simulink model "SAFECOPYFOC_Motor_Control_Hardware"  (R2025b)
settings: Solver=FixedStepDiscrete  StartTime=0.0  StopTime=inf  FixedStep=50e-6  MaxStep=1e-4  RelTol=1e-3  EnableMultiTasking=on
values from neighbouring files (symbols this model uses):
  Ki_d = R   * omega_c    [VirtualSpeedDynoParams.m]
  Ki_q = R   * omega_c    [VirtualSpeedDynoParams.m]
  Kp_d = L_d * omega_c    [VirtualSpeedDynoParams.m]
  Kp_q = L_q * omega_c    [VirtualSpeedDynoParams.m]
  L_d = motor.L_phase_H    [VirtualSpeedDynoParams.m]
  L_q = motor.L_phase_H    [VirtualSpeedDynoParams.m]
  lambda = motor.lambda_Wb    [VirtualSpeedDynoParams.m]
  p = motor.pole_pairs    [VirtualSpeedDynoParams.m]
  V_bat = motor.bus_voltage_V    [VirtualSpeedDynoParams.m]
undefined symbols (not defined in the file or in its folder): bit, Down, GPTRIP1SEL, GPTRIP2SEL, target, TZ1, TZ2, Up
libraries: c2802xlib x5, c280xlib x3, slpidlib x3, c2806xlib x2, eeTransforms x2, simulink x1

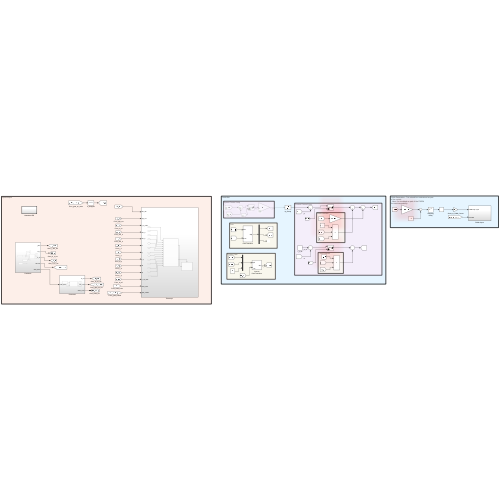
[thumbnail: Simulink's stored preview of the top-level diagram]
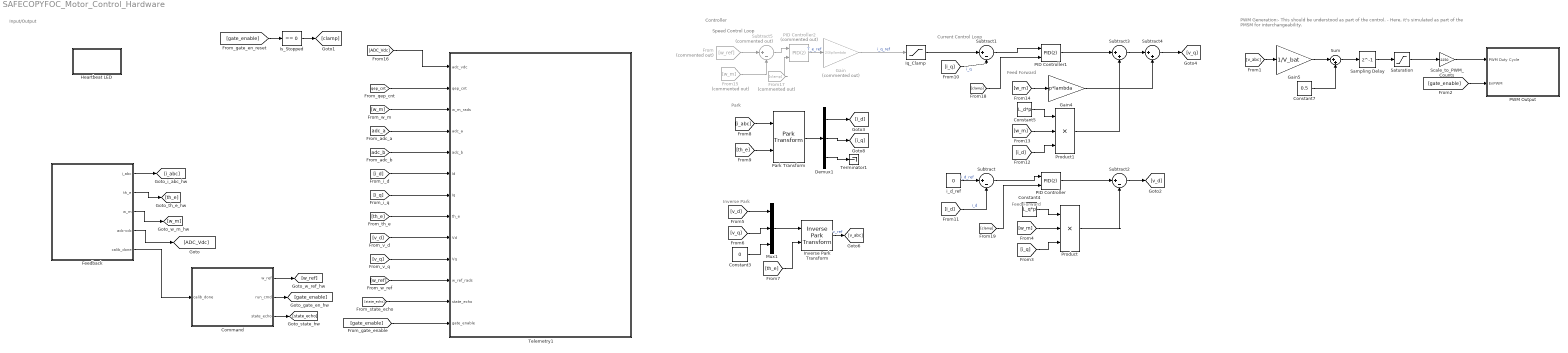
== system SAFECOPYFOC_Motor_Control_Hardware ==
  note: Feed Forward
  note: Feed Forward
  note: Current Control Loop
  note: Speed Control Loop
  note: Input/Output
  note: Park
  note: Inverse Park
  note: PWM Generation:- This should be understood as part
      | of the control.
      | - Here, it's simulated as part of the PMSM
      | for interchangeability.
  note: Controller
  Command : Subsystem
  Constant3 : Constant  Value=0  OutDataTypeStr=single
  Constant4 : Constant  Value=L_q*p  OutDataTypeStr=single
  Constant5 : Constant  Value=L_d*p  OutDataTypeStr=single
  Constant7 : Constant  Value=0.5  OutDataTypeStr=single
  Demux1 : Demux  Outputs=3
  Feedback : Subsystem
  From : From  Commented=on  GotoTag=w_ref
  From15 : From  Commented=on  GotoTag=w_m
  From17 : From  Commented=on  GotoTag=clamp
  Gain : Gain  Commented=on  Gain=2/3/p/lambda
  Gain4 : Gain  Gain=p*lambda
  Gain5 : Gain  Gain=1/V_bat
  Heartbeat LED : Subsystem  TreatAsAtomicUnit=on
  Inverse Park Transform : eeTransforms/Inverse Park Transform  AxisAlignment=D-axis  PowerInvariant=off
  Iq_Clamp : Saturate
  Is_Stopped : simulink/Logic and Bit Operations/Compare To Zero  relop===  OutDataTypeStr=boolean
  Mux1 : Mux  Inputs=3
  PID Controller : slpidlib/PID Controller  Controller=PID  Form=Parallel  TimeDomain=Discrete-time  UseExternalTs=off  SampleTime=50e-6  IntegratorMethod=Forward Euler  FilterMethod=Forward Euler  ControllerParametersSource=internal  P=Kp_d  I=Ki_d  UseKiTs=off  D=0  UseExternalDerivativeSource=off  N=100  UseFilter=on  TunerSelectOption=Transfer Function Based (PID Tuner App)  InitialConditionSource=internal  InitialConditionForIntegrator=0  InitialConditionForFilter=0  DifferentiatorICPrevScaledInput=0  ExternalReset=level  TrackingMode=off  Kt=1  LimitOutput=on  SatLimitsSource=internal  UpperSaturationLimit=V_bat/sqrt(3)  LowerSaturationLimit=-(V_bat/sqrt(3))  LinearizeAsGain=on  AntiWindupMode=clamping  Kb=1  LimitIntegrator=off  UpperIntegratorSaturationLimit=inf  LowerIntegratorSaturationLimit=-inf  POutMin=[]  POutMax=[]  IOutMin=[]  IOutMax=[]  DOutMin=[]  DOutMax=[]  NOutMin=[]  NOutMax=[]  SumOutMin=[]  SumOutMax=[]  SaturationOutMin=[]  SaturationOutMax=[]  PParamMin=[]  PParamMax=[]  IParamMin=[]  IParamMax=[]  DParamMin=[]  DParamMax=[]  NParamMin=[]  NParamMax=[]  KbParamMin=[]  KbParamMax=[]  KtParamMin=[]  KtParamMax=[]  KbOutMin=[]  KbOutMax=[]  KtOutMin=[]  KtOutMax=[]  IntegratorOutMin=[]  IntegratorOutMax=[]  FilterOutMin=[]  FilterOutMax=[]  SumI1OutMin=[]  SumI1OutMax=[]  SumI2OutMin=[]  SumI2OutMax=[]  SumI3OutMin=[]  SumI3OutMax=[]  SumI4OutMin=[]  SumI4OutMax=[]  SumDOutMin=[]  SumDOutMax=[]  DifferentiatorOutMin=[]  DifferentiatorOutMax=[]  FilterDiffOutCoefMin=[]  FilterDiffOutCoefMax=[]  ReciprocalOutMin=[]  ReciprocalOutMax=[]  SumDenOutMin=[]  SumDenOutMax=[]  SumNumOutMin=[]  SumNumOutMax=[]  DivideOutMin=[]  DivideOutMax=[]  UdiffTsProdOutMin=[]  UdiffTsProdOutMax=[]  NTsProdOutMin=[]  NTsProdOutMax=[]  UintegralTsProdOutMin=[]  UintegralTsProdOutMax=[]  UngainTsProdOutMin=[]  UngainTsProdOutMax=[]  ClampingZeroOutDataTypeStr=Inherit: Inherit via back propagation  ClampingZeroOutMin=[]  ClampingZeroOutMax=[]  FilterDenConstantOutDataTypeStr=Inherit: Inherit via back propagation  FilterDenConstantOutMin=[]  FilterDenConstantOutMax=[]  PCopyOutDataTypeStr=Inherit: Inherit via back propagation  PCopyOutMin=[]  PCopyOutMax=[]  NCopyOutDataTypeStr=Inherit: Inherit via back propagation  NCopyOutMin=[]  NCopyOutMax=[]  IntegratorContinuousStateAttributes=''  IntegratorStateMustResolveToSignalObject=off  IntegratorRTWStateStorageClass=Auto  FilterContinuousStateAttributes=''  FilterStateMustResolveToSignalObject=off  FilterRTWStateStorageClass=Auto  ParallelPVariant=InternalParameters  IdealPVariant=Disabled  IVariant=InternalParameters  DVariant=InternalParameters  IntegratorVariant=Discrete  SatVariant=Enabled  AWVariant=DiscClampingParallel  PCopyVariant=Disabled  TRVariant=Disabled  FdbkBlocksVariant=Forward  IdealPFdbkVariant=Disabled  SatFdbkVariant=Disabled  DerivativeFilterVariant=ForwardEulerFilter  NVariant=InternalParameters  NCopyVariant=Disabled  FilterICVariant=InternalICsFilter  IntegratorICVariant=InternalICs  ExternalResetVariant=ExternalReset  TRSumVariant=Passthrough  SumFdbkVariant=Disabled  SumVariant=Sum_PID  TsampFilterVariant=InternalTs  TsampNgainVariant=Passthrough  TsampIntegralVariant=Disabled_SignalSpec  ExternalSaturationOutDataTypeStr=Inherit: Same as second input  DerivativeSourceVariant=ErrorSignal  PreIntVariant=InternalPreInt
  PID Controller1 : slpidlib/PID Controller  Controller=PID  Form=Parallel  TimeDomain=Discrete-time  UseExternalTs=off  SampleTime=50e-6  IntegratorMethod=Forward Euler  FilterMethod=Forward Euler  ControllerParametersSource=internal  P=Kp_q  I=Ki_q  UseKiTs=off  D=0  UseExternalDerivativeSource=off  N=100  UseFilter=on  TunerSelectOption=Transfer Function Based (PID Tuner App)  InitialConditionSource=internal  InitialConditionForIntegrator=0  InitialConditionForFilter=0  DifferentiatorICPrevScaledInput=0  ExternalReset=level  TrackingMode=off  Kt=1  LimitOutput=on  SatLimitsSource=internal  UpperSaturationLimit=V_bat/sqrt(3)  LowerSaturationLimit=-(V_bat/sqrt(3))  LinearizeAsGain=on  AntiWindupMode=clamping  Kb=1  LimitIntegrator=off  UpperIntegratorSaturationLimit=inf  LowerIntegratorSaturationLimit=-inf  POutMin=[]  POutMax=[]  IOutMin=[]  IOutMax=[]  DOutMin=[]  DOutMax=[]  NOutMin=[]  NOutMax=[]  SumOutMin=[]  SumOutMax=[]  SaturationOutMin=[]  SaturationOutMax=[]  PParamMin=[]  PParamMax=[]  IParamMin=[]  IParamMax=[]  DParamMin=[]  DParamMax=[]  NParamMin=[]  NParamMax=[]  KbParamMin=[]  KbParamMax=[]  KtParamMin=[]  KtParamMax=[]  KbOutMin=[]  KbOutMax=[]  KtOutMin=[]  KtOutMax=[]  IntegratorOutMin=[]  IntegratorOutMax=[]  FilterOutMin=[]  FilterOutMax=[]  SumI1OutMin=[]  SumI1OutMax=[]  SumI2OutMin=[]  SumI2OutMax=[]  SumI3OutMin=[]  SumI3OutMax=[]  SumI4OutMin=[]  SumI4OutMax=[]  SumDOutMin=[]  SumDOutMax=[]  DifferentiatorOutMin=[]  DifferentiatorOutMax=[]  FilterDiffOutCoefMin=[]  FilterDiffOutCoefMax=[]  ReciprocalOutMin=[]  ReciprocalOutMax=[]  SumDenOutMin=[]  SumDenOutMax=[]  SumNumOutMin=[]  SumNumOutMax=[]  DivideOutMin=[]  DivideOutMax=[]  UdiffTsProdOutMin=[]  UdiffTsProdOutMax=[]  NTsProdOutMin=[]  NTsProdOutMax=[]  UintegralTsProdOutMin=[]  UintegralTsProdOutMax=[]  UngainTsProdOutMin=[]  UngainTsProdOutMax=[]  ClampingZeroOutDataTypeStr=Inherit: Inherit via back propagation  ClampingZeroOutMin=[]  ClampingZeroOutMax=[]  FilterDenConstantOutDataTypeStr=Inherit: Inherit via back propagation  FilterDenConstantOutMin=[]  FilterDenConstantOutMax=[]  PCopyOutDataTypeStr=Inherit: Inherit via back propagation  PCopyOutMin=[]  PCopyOutMax=[]  NCopyOutDataTypeStr=Inherit: Inherit via back propagation  NCopyOutMin=[]  NCopyOutMax=[]  IntegratorContinuousStateAttributes=''  IntegratorStateMustResolveToSignalObject=off  IntegratorRTWStateStorageClass=Auto  FilterContinuousStateAttributes=''  FilterStateMustResolveToSignalObject=off  FilterRTWStateStorageClass=Auto  ParallelPVariant=InternalParameters  IdealPVariant=Disabled  IVariant=InternalParameters  DVariant=InternalParameters  IntegratorVariant=Discrete  SatVariant=Enabled  AWVariant=DiscClampingParallel  PCopyVariant=Disabled  TRVariant=Disabled  FdbkBlocksVariant=Forward  IdealPFdbkVariant=Disabled  SatFdbkVariant=Disabled  DerivativeFilterVariant=ForwardEulerFilter  NVariant=InternalParameters  NCopyVariant=Disabled  FilterICVariant=InternalICsFilter  IntegratorICVariant=InternalICs  ExternalResetVariant=ExternalReset  TRSumVariant=Passthrough  SumFdbkVariant=Disabled  SumVariant=Sum_PID  TsampFilterVariant=InternalTs  TsampNgainVariant=Passthrough  TsampIntegralVariant=Disabled_SignalSpec  ExternalSaturationOutDataTypeStr=Inherit: Same as second input  DerivativeSourceVariant=ErrorSignal  PreIntVariant=InternalPreInt
  PID Controller2 : slpidlib/PID Controller  Commented=on  Controller=PID  Form=Parallel  TimeDomain=Discrete-time  UseExternalTs=off  SampleTime=50e-6  IntegratorMethod=Forward Euler  FilterMethod=Forward Euler  ControllerParametersSource=internal  P=2.5  I=1.5  UseKiTs=off  D=0  UseExternalDerivativeSource=off  N=100  UseFilter=on  TunerSelectOption=Transfer Function Based (PID Tuner App)  InitialConditionSource=internal  InitialConditionForIntegrator=0  InitialConditionForFilter=0  DifferentiatorICPrevScaledInput=0  ExternalReset=level  TrackingMode=off  Kt=1  LimitOutput=on  SatLimitsSource=internal  UpperSaturationLimit=60  LowerSaturationLimit=-60  LinearizeAsGain=on  AntiWindupMode=clamping  Kb=1  LimitIntegrator=off  UpperIntegratorSaturationLimit=inf  LowerIntegratorSaturationLimit=-inf  POutMin=[]  POutMax=[]  IOutMin=[]  IOutMax=[]  DOutMin=[]  DOutMax=[]  NOutMin=[]  NOutMax=[]  SumOutMin=[]  SumOutMax=[]  SaturationOutMin=[]  SaturationOutMax=[]  PParamMin=[]  PParamMax=[]  IParamMin=[]  IParamMax=[]  DParamMin=[]  DParamMax=[]  NParamMin=[]  NParamMax=[]  KbParamMin=[]  KbParamMax=[]  KtParamMin=[]  KtParamMax=[]  KbOutMin=[]  KbOutMax=[]  KtOutMin=[]  KtOutMax=[]  IntegratorOutMin=[]  IntegratorOutMax=[]  FilterOutMin=[]  FilterOutMax=[]  SumI1OutMin=[]  SumI1OutMax=[]  SumI2OutMin=[]  SumI2OutMax=[]  SumI3OutMin=[]  SumI3OutMax=[]  SumI4OutMin=[]  SumI4OutMax=[]  SumDOutMin=[]  SumDOutMax=[]  DifferentiatorOutMin=[]  DifferentiatorOutMax=[]  FilterDiffOutCoefMin=[]  FilterDiffOutCoefMax=[]  ReciprocalOutMin=[]  ReciprocalOutMax=[]  SumDenOutMin=[]  SumDenOutMax=[]  SumNumOutMin=[]  SumNumOutMax=[]  DivideOutMin=[]  DivideOutMax=[]  UdiffTsProdOutMin=[]  UdiffTsProdOutMax=[]  NTsProdOutMin=[]  NTsProdOutMax=[]  UintegralTsProdOutMin=[]  UintegralTsProdOutMax=[]  UngainTsProdOutMin=[]  UngainTsProdOutMax=[]  ClampingZeroOutDataTypeStr=Inherit: Inherit via back propagation  ClampingZeroOutMin=[]  ClampingZeroOutMax=[]  FilterDenConstantOutDataTypeStr=Inherit: Inherit via back propagation  FilterDenConstantOutMin=[]  FilterDenConstantOutMax=[]  PCopyOutDataTypeStr=Inherit: Inherit via back propagation  PCopyOutMin=[]  PCopyOutMax=[]  NCopyOutDataTypeStr=Inherit: Inherit via back propagation  NCopyOutMin=[]  NCopyOutMax=[]  IntegratorContinuousStateAttributes=''  IntegratorStateMustResolveToSignalObject=off  IntegratorRTWStateStorageClass=Auto  FilterContinuousStateAttributes=''  FilterStateMustResolveToSignalObject=off  FilterRTWStateStorageClass=Auto  ParallelPVariant=InternalParameters  IdealPVariant=Disabled  IVariant=InternalParameters  DVariant=InternalParameters  IntegratorVariant=Discrete  SatVariant=Enabled  AWVariant=DiscClampingParallel  PCopyVariant=Disabled  TRVariant=Disabled  FdbkBlocksVariant=Forward  IdealPFdbkVariant=Disabled  SatFdbkVariant=Disabled  DerivativeFilterVariant=ForwardEulerFilter  NVariant=InternalParameters  NCopyVariant=Disabled  FilterICVariant=InternalICsFilter  IntegratorICVariant=InternalICs  ExternalResetVariant=ExternalReset  TRSumVariant=Passthrough  SumFdbkVariant=Disabled  SumVariant=Sum_PID  TsampFilterVariant=InternalTs  TsampNgainVariant=Passthrough  TsampIntegralVariant=Disabled_SignalSpec  ExternalSaturationOutDataTypeStr=Inherit: Same as second input  DerivativeSourceVariant=ErrorSignal  PreIntVariant=InternalPreInt
  PWM Output : Subsystem
  Park Transform : eeTransforms/Park Transform  AxisAlignment=D-axis  PowerInvariant=off
  Product : Product  Inputs=3
  Product1 : Product  Inputs=3
  Sampling Delay : Delay  DelayLength=1
  Saturation : Saturate  UpperLimit=1  LowerLimit=0
  Scale_to_PWM_Counts : Gain  Gain=2250
  Subtract : Sum  Inputs=|+-
  Subtract1 : Sum  Inputs=|+-
  Subtract2 : Sum  Inputs=|+-
  Subtract3 : Sum  Inputs=|++
  Subtract4 : Sum  Inputs=|++
  Subtract5 : Sum  Commented=on  Inputs=|+-
  Sum : Sum  Inputs=|++
  Telemetry1 : Subsystem
  Terminator1 : Terminator
  i_d_ref : Constant  Value=0  OutDataTypeStr=single
  wires:
  [qep_cnt] -> Telemetry1/2(qep_cnt)
  [w_m] -> Telemetry1/3(w_m_rads)
  [adc_a] -> Telemetry1/4(adc_a)
  [adc_b] -> Telemetry1/5(adc_b)
  [i_d] -> Telemetry1/6(Id)
  [i_q] -> Telemetry1/7(Iq)
  [th_e] -> Telemetry1/8(th_e)
  [v_d] -> Telemetry1/9(Vd)
  [v_q] -> Telemetry1/10(Vq)
  [w_ref] -> Telemetry1/11(w_ref_rads)
  [state_echo] -> Telemetry1/12(state_echo)
  [gate_enable] -> Telemetry1/13(gate_enable)
  Command/1(w_ref) -> [w_ref]
  Command/2(run_cmd) -> [gate_enable]
  Command/3(state_echo) -> [state_echo]
  Feedback/5(calib_done) -> Command/1(calib_done)
  Feedback/3(w_m) -> [w_m]
  Feedback/2(th_e) -> [th_e]
  Feedback/1(i_abc) -> [i_abc]
  From/1 -> Subtract5/1
  From15/1 -> Subtract5/2
  Subtract5/1 -> PID Controller2/1
  PID Controller2/1 -> Gain/1  "T_e_ref"
  Gain/1 -> Iq_Clamp/1  "i_q_ref"
  Iq_Clamp/1 -> Subtract1/1
  [i_q] -> Subtract1/2  "i_q"
  Subtract1/1 -> PID Controller1/1
  PID Controller1/1 -> Subtract3/1
  Product1/1 -> Subtract3/2
  [w_m] -> Gain4/1
  Constant5/1 -> Product1/1
  [w_m] -> Product1/2
  [i_d] -> Product1/3
  Gain4/1 -> Subtract4/2
  Subtract3/1 -> Subtract4/1
  Subtract4/1 -> [v_q]
  [v_abc] -> Gain5/1
  Gain5/1 -> Sum/1
  Constant7/1 -> Sum/2
  Sum/1 -> Sampling Delay/1
  Sampling Delay/1 -> Saturation/1
  Saturation/1 -> Scale_to_PWM_Counts/1
  Scale_to_PWM_Counts/1 -> PWM Output/1(PWM Duty Cycle)
  [gate_enable] -> PWM Output/2(EnPWM)
  i_d_ref/1 -> Subtract/1  "i_d_ref"
  [i_d] -> Subtract/2  "i_d"
  Subtract/1 -> PID Controller/1
  PID Controller/1 -> Subtract2/1
  Product/1 -> Subtract2/2
  Subtract2/1 -> [v_d]
  Constant4/1 -> Product/1
  [w_m] -> Product/2
  [i_q] -> Product/3
  Inverse Park Transform/1 -> [v_abc]  "v_ref"
  Mux1/1 -> Inverse Park Transform/1
  [th_e] -> Inverse Park Transform/2
  Constant3/1 -> Mux1/3
  [v_q] -> Mux1/2
  [v_d] -> Mux1/1
  [th_e] -> Park Transform/2
  [i_abc] -> Park Transform/1
  Demux1/1 -> [i_d]
  Demux1/2 -> [i_q]
  Demux1/3 -> Terminator1/1
  Park Transform/1 -> Demux1/1
  Feedback/4(adc-vdc) -> [ADC_Vdc]
  [ADC_Vdc] -> Telemetry1/1(adc_vdc)
  [gate_enable] -> Is_Stopped/1
  Is_Stopped/1 -> [clamp]
  From17/1 -> PID Controller2/2
  [clamp] -> PID Controller1/2
  [clamp] -> PID Controller/2

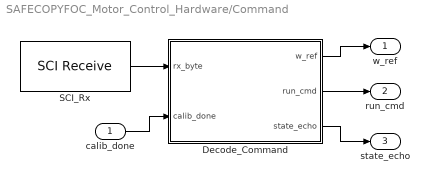
== system SAFECOPYFOC_Motor_Control_Hardware/Command ==
  calib_done : Inport
  Decode_Command : MATLAB Function  TreatAsAtomicUnit=on
  SCI_Rx : c280xlib/SCI Receive  sciModule=A  dataHead=''  headerCheckMaxCount=16  dataTail=''  dataType=uint8  dataLenOptions=Length via dialog  dataDim=1  maxDataLength=1  initValue=0  errOption=Output custom value  errValue=0  sampleTime=-1  blockingMode=off  timeOut=0.019444  outputStatus=off
  w_ref : Outport
  run_cmd : Outport  Port=2
  state_echo : Outport  Port=3
  wires:
  Decode_Command/3(state_echo) -> state_echo/1
  SCI_Rx/1 -> Decode_Command/1(rx_byte)
  calib_done/1 -> Decode_Command/2(calib_done)
  Decode_Command/1(w_ref) -> w_ref/1
  Decode_Command/2(run_cmd) -> run_cmd/1

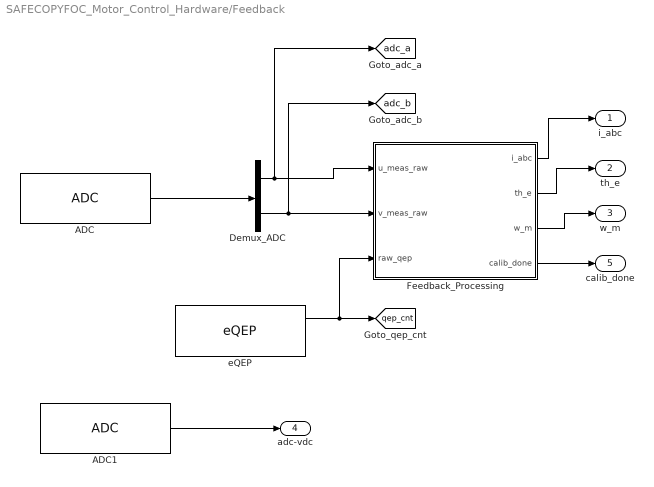
== system SAFECOPYFOC_Motor_Control_Hardware/Feedback ==
  ADC : c2802xlib/ADC  blkParamProc=C2000  ADCModule=1  samplingMode=Simultaneous sample mode  ADCResolution=12-bit (Single-ended input)  ADC29xResolution=12-bit  ADCMode=Single-ended input  useSOC1=SOC0  useSOC2=SOC0_SOC1  SOCAcquisitionWindow=7  SOCTriggerSource=Software  SOCInterruptTrigger=No ADCINT  Ts=-1  dType=uint16  postInterrupt=on  interruptSel=ADCINT1  ADCINTContinuous=on  endma=off  chdma=1  conv1=ADCINA0  conv2=ADCINA3 and ADCINB3  conv1_Type4=ADCIN0  conv2_Type4=ADCIN0 and ADCIN1
  ADC1 : c2802xlib/ADC  blkParamProc=C2000  ADCModule=1  samplingMode=Simultaneous sample mode  ADCResolution=12-bit (Single-ended input)  ADC29xResolution=12-bit  ADCMode=Single-ended input  useSOC1=SOC2  useSOC2=SOC2_SOC3  SOCAcquisitionWindow=7  SOCTriggerSource=Software  SOCInterruptTrigger=No ADCINT  Ts=-1  dType=uint16  postInterrupt=off  interruptSel=ADCINT1  ADCINTContinuous=on  endma=off  chdma=1  conv1=ADCINB7  conv2=ADCINA1 and ADCINB1  conv1_Type4=ADCIN0  conv2_Type4=ADCIN0 and ADCIN1
  Demux_ADC : Demux  Outputs=2
  Feedback_Processing : MATLAB Function  TreatAsAtomicUnit=on
  eQEP : c280xlib/eQEP  useModule=eQEP1  pcInputmode=Quadrature-count  externalClockrate=2x resolution: Count the rising/falling edge  swapPolarityselection=Clockwise  qdfOutputport=off  qapPolarityselection=off  qbpPolarityselection=off  qipPolarityselection=off  qspPolarityselection=off  igatePolarityselection=off  sampleTime=-1  pcOutputport=on  pcMaximumvalue=4*1024 - 1  indexInitializationcheck=off  indexInitializationevent=Falling edge  strobeInitializationcheck=off  strobeInitializationevent=Rising edge  softwareInitializationcheck=off  softwareInitializationsource=Set to init value at start up  softwareInitializationmode=on  pcInitialvalue=0  pcResetmode=Reset on the first index event  ieloutputport=on  indexEventlatch=Rising edge  seloutputport=off  strobeEventlatch=Rising edge  pcefOutputport=off  enableEqepcapture=off  qctmrOutputport=off  qcprdOutputport=off  captureTimerprescaler=128  upEventprescaler=128  overflowErrorflag=off  directionErrorflag=off  captureTimerposition=On position counter read  unitTimerperiod=100000000  captureTimerlatch=off  capturePeriodlatch=off  positionCounterlatch=off  soenPolarityselection=off  spselPolarityselection=Index pin is used for sync output  compareValuesource=Specify via dialog  shadowMode=Load on QPOSCNT=0  compareValue=4294967295  syncOutputwidth=1  polaritySyncoutput=Active high  watchdogEnable=off  watchdogTimer=65535  outport1Datatype=auto  outport2Datatype=auto  outport3Datatype=auto  outport4Datatype=auto  outport5Datatype=auto  outport6Datatype=auto  outport7Datatype=auto  outport8Datatype=auto  outport9Datatype=auto  outport10Datatype=auto  outport11Datatype=auto  outport12Datatype=auto  eqepinterrupt_pce=off  eqepinterrupt_qpe=off  eqepinterrupt_qdc=off  eqepinterrupt_wto=off  eqepinterrupt_pcu=off  eqepinterrupt_pco=off  eqepinterrupt_pcr=off  eqepinterrupt_pcm=off  eqepinterrupt_sel=off  eqepinterrupt_iel=off  eqepinterrupt_uto=off  pheOutputport=off  watchdogOutputport=off  outport13Datatype=auto  outport14Datatype=auto
  i_abc : Outport
  th_e : Outport  Port=2
  w_m : Outport  Port=3
  adc-vdc : Outport  Port=4
  calib_done : Outport  Port=5
  tag scope: adc_a=global, adc_b=global, qep_cnt=global
  wires:
  Demux_ADC/1 -> Feedback_Processing/1(u_meas_raw), [adc_a]
  ADC/1 -> Demux_ADC/1
  Feedback_Processing/2(th_e) -> th_e/1
  eQEP/1 -> [qep_cnt], Feedback_Processing/3(raw_qep)
  Demux_ADC/2 -> Feedback_Processing/2(v_meas_raw), [adc_b]
  Feedback_Processing/1(i_abc) -> i_abc/1
  Feedback_Processing/4(calib_done) -> calib_done/1
  Feedback_Processing/3(w_m) -> w_m/1
  ADC1/1 -> adc-vdc/1

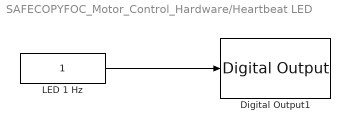
== system SAFECOPYFOC_Motor_Control_Hardware/Heartbeat LED ==
  Digital Output1 : c2806xlib/Digital Output  GPIO_Number=GPIO32~GPIO39  GPIO_Bit0=off  GPIO_BIT0_Toggle=off  GPIO_Bit1=off  GPIO_BIT1_Toggle=off  GPIO_Bit2=on  GPIO_BIT2_Toggle=on  GPIO_Bit3=off  GPIO_BIT3_Toggle=off  GPIO_Bit4=off  GPIO_BIT4_Toggle=off  GPIO_Bit5=off  GPIO_BIT5_Toggle=off  GPIO_Bit6=off  GPIO_BIT6_Toggle=off  GPIO_Bit7=off  GPIO_BIT7_Toggle=off
  LED 1 Hz : Constant  OutDataTypeStr=uint16  SampleTime=0.5
  wires:
  LED 1 Hz/1 -> Digital Output1/1

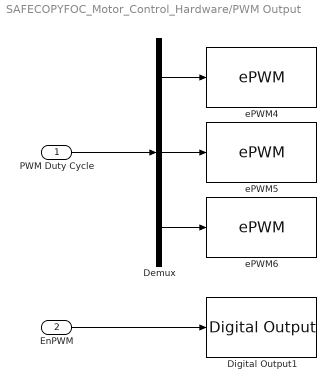
== system SAFECOPYFOC_Motor_Control_Hardware/PWM Output ==
  PWM Duty Cycle : Inport
  EnPWM : Inport  Port=2
  Demux : Demux  Outputs=3
  Digital Output1 : c2806xlib/Digital Output  GPIO_Number=GPIO50~GPIO55  GPIO_Bit0=off  GPIO_BIT0_Toggle=off  GPIO_Bit1=off  GPIO_BIT1_Toggle=off  GPIO_Bit2=on  GPIO_BIT2_Toggle=off  GPIO_Bit3=off  GPIO_BIT3_Toggle=off  GPIO_Bit4=off  GPIO_BIT4_Toggle=off  GPIO_Bit5=off  GPIO_BIT5_Toggle=off  GPIO_Bit6=off  GPIO_BIT6_Toggle=off  GPIO_Bit7=off  GPIO_BIT7_Toggle=off
  ePWM4 : c2802xlib/ePWM  PwmType=C2000  useModule=ePWM4  ePWMxLINKTBPRD=Not Linked  periodUnits=Clock cycles  timerSource=Specify via dialog  timerPeriod_clk=2250  timerPeriod_sec=64000  tbshadow=Counter equals to zero  countingMode=Up-Down  phaseActiveEnable=Disable  phaseDirection=Count down after sync  phaseActive=0  synchronizationEnable=off  dcaevt1Sync=off  dcbevt1Sync=off  synchronizationOption=Counter equals to zero (CTR=Zero)  dcbevt1SyncOut=off  dcaevt1SyncOut=off  cmpdSyncOut=off  cmpcSyncOut=off  cmpbSyncOut=off  zeroSyncOut=on  swfSyncOut=off  perSynchronizationOption=Counter equals to period (CTR=PRD)  clockPrescale=1  HSclockPrescale=1  enswap=off  ePWMxAStatus=on  ePWMxAactionLogic1=Do nothing  ePWMxAactionLogic2=Do nothing  ePWMxAactionLogic3=Clear  ePWMxAactionLogic4=Set  ePWMxAactionLogic5=Do nothing  ePWMxAactionLogic6=Do nothing  ePWMxACSFenable=off  ePWMxACSFvalue=Forcing disable  ePWMxASFreload=Zero  ePWMxBStatus=off  ePWMxBactionLogic1=Do nothing  ePWMxBactionLogic2=Set  ePWMxBactionLogic3=Do nothing  ePWMxBactionLogic4=Do nothing  ePWMxBactionLogic5=Clear  ePWMxBactionLogic6=Do nothing  ePWMxBCSFenable=off  ePWMxBCSFvalue=Forcing disable  ePWMxBSFreload=Zero  ePWNxBOutWay=off  ePWMxLINKCMPA=Not Linked  CMPAUnits=Clock cycles  CMPASource=Input port  CMPAValue_per=32000  CMPAValue_clk=floor(target.PWM_Counter_Period/2+1)  enCMPAshadow=Counter equals to zero (CTR=Zero)  ePWMxLINKCMPB=Not Linked  CMPBUnits=Clock cycles  CMPBSource=Specify via dialog  CMPBValue_per=50  CMPBValue_clk=floor(target.PWM_Counter_Period/2+1)  enCMPBshadow=Counter equals to zero (CTR=Zero)  ePWMxLINKCMPC=Not Linked  CMPCUnits=Clock cycles  CMPCSource=Specify via dialog  CMPCValue_per=50  CMPCValue_clk=32000  enCMPCshadow=Counter equals to zero (CTR=Zero)  ePWMxLINKCMPD=Not Linked  CMPDUnits=Clock cycles  CMPDSource=Specify via dialog  CMPDValue_per=50  CMPDValue_clk=32000  enCMPDshadow=Counter equals to zero (CTR=Zero)  enableDBePWMxA=on  enableDBePWMxB=on  enhalfcycle=off  DBpolarity=Active high complementary (AHC)  DBedgeDelay=Positive  DBSource_ePWMxA=ePWMxA  DBSource_ePWMxB=ePWMxA  DBPeriodUnits=Clock cycles  DBperiodSource=Specify via dialog  REDperiod=5  FEDperiod=5  REDperiod_sec=0  FEDperiod_sec=0  LoadModeDBRED=Immediate without using shadow  LoadModeDBFED=Immediate without using shadow  adcstartModuleA=on  adcrequestEventA=First event  adcstartEventA=Counter equals to period (CTR=PRD)  adcstartEventA_type2=Digital Compare Module A Event 1 start of conversion (DCAEVT1.soc)  adcstartModuleB=off  adcrequestEventB=First event  adcstartEventB=Counter equals to zero (CTR=Zero)  adcstartEventB_type2=Counter equals to zero (CTR=Zero)  intEn=off  intPrd=First event  intSel=Counter equals to zero (CTR=Zero)  intSel_type2=Counter equals to zero (CTR=Zero)  hrpe=off  enHRPWM=off  HRPWM_LoadMode=Counter equals to period (CTR=PRD)  HRPWM_CTLMode=Duty or Period control mode  HRPWM_EDGMode=Both edge  hrpeb=off  enHRPWMB=off  HRPWM_LoadModeB=Counter equals to zero (CTR=ZERO)  HRPWM_CTLModeB=Duty or Period control mode  HRPWM_EDGModeB=Both edge  enHRDBRED=off  enHRDBFED=off  enSFO=on  enautoconv=on  chopperEnable=off  chopperFrequency=1  chopperFirstwidth=1  chopperDuty=12.5%  tripZonesource=Specify via dialog  tzselOSHT1=off  tzselOSHT2=off  tzselOSHT3=off  tzselOSHT4=off  tzselOSHT5=off  tzselOSHT6=off  tzselOSHDCAEV1=off  tzselOSHDCBEV1=off  tzselCBC1=off  tzselCBC2=off  tzselCBC3=off  tzselCBC4=off  tzselCBC5=off  tzselCBC6=off  tzselCBCDCAEV2=off  tzselCBCDCBEV2=off  enTzOstIntr=off  enTzCbcIntr=off  enTzDCAEVT1Intr=off  enTzDCAEVT2Intr=off  enTzDCBEVT1Intr=off  enTzDCBEVT2Intr=off  tzclrCBCLatch=Counter equals to zero (CTR=Zero)  ePWMxAforced=No action  ePWMxBforced=No action  DCAEVT1forced=No action  DCBEVT1forced=No action  DCAEVT2forced=No action  DCBEVT2forced=No action  dcah=Trip Zone 1 input (TZ1)  dcal=Trip Zone 2 input (TZ2)  dcbh=Trip Zone 1 input (TZ1)  dcbl=Trip Zone 2 input (TZ2)  dcah_type2=GPTRIP1SEL/(TZ1)  dcal_type2=GPTRIP2SEL/(TZ2)  dcbh_type2=GPTRIP1SEL/(TZ1)  dcbl_type2=GPTRIP2SEL/(TZ2)  gendcaevt1=Event disabled  gendcaevt2=Event disabled  gendcbevt1=Event disabled  gendcbevt2=Event disabled  dcaevt1src=DCAEVT1 with sync  dcaevt2src=DCAEVT2 with sync  dcbevt1src=DCBEVT1 with sync  dcbevt2src=DCBEVT2 with sync  pulsesel=Counter equals to zero (CTR=Zero)  blankinv=off  blankoffset=0  blankwidth=0  evsrcsel=Filtered version of DCAEVT1 (DCAEVT1FILT)  encape=off
  ePWM5 : c2802xlib/ePWM  PwmType=C2000  useModule=ePWM5  ePWMxLINKTBPRD=Not Linked  periodUnits=Clock cycles  timerSource=Specify via dialog  timerPeriod_clk=2250  timerPeriod_sec=64000  tbshadow=Counter equals to zero  countingMode=Up-Down  phaseActiveEnable=Set counter to phase value specified via dialog  phaseDirection=Count up after sync  phaseActive=0  synchronizationEnable=off  dcaevt1Sync=off  dcbevt1Sync=off  synchronizationOption=Pass through (EPWMxSYNCI or SWFSYNC)  dcbevt1SyncOut=off  dcaevt1SyncOut=off  cmpdSyncOut=off  cmpcSyncOut=off  cmpbSyncOut=off  zeroSyncOut=off  swfSyncOut=on  perSynchronizationOption=Counter equals to period (CTR=PRD)  clockPrescale=1  HSclockPrescale=1  enswap=off  ePWMxAStatus=on  ePWMxAactionLogic1=Do nothing  ePWMxAactionLogic2=Do nothing  ePWMxAactionLogic3=Clear  ePWMxAactionLogic4=Set  ePWMxAactionLogic5=Do nothing  ePWMxAactionLogic6=Do nothing  ePWMxACSFenable=off  ePWMxACSFvalue=Forcing disable  ePWMxASFreload=Zero  ePWMxBStatus=off  ePWMxBactionLogic1=Do nothing  ePWMxBactionLogic2=Set  ePWMxBactionLogic3=Do nothing  ePWMxBactionLogic4=Do nothing  ePWMxBactionLogic5=Clear  ePWMxBactionLogic6=Do nothing  ePWMxBCSFenable=off  ePWMxBCSFvalue=Forcing disable  ePWMxBSFreload=Zero  ePWNxBOutWay=off  ePWMxLINKCMPA=Not Linked  CMPAUnits=Clock cycles  CMPASource=Input port  CMPAValue_per=32000  CMPAValue_clk=floor(target.PWM_Counter_Period/2+1)  enCMPAshadow=Counter equals to zero (CTR=Zero)  ePWMxLINKCMPB=Not Linked  CMPBUnits=Clock cycles  CMPBSource=Specify via dialog  CMPBValue_per=50  CMPBValue_clk=floor(target.PWM_Counter_Period/2+1)  enCMPBshadow=Counter equals to zero (CTR=Zero)  ePWMxLINKCMPC=Not Linked  CMPCUnits=Clock cycles  CMPCSource=Specify via dialog  CMPCValue_per=50  CMPCValue_clk=32000  enCMPCshadow=Counter equals to zero (CTR=Zero)  ePWMxLINKCMPD=Not Linked  CMPDUnits=Clock cycles  CMPDSource=Specify via dialog  CMPDValue_per=50  CMPDValue_clk=32000  enCMPDshadow=Counter equals to zero (CTR=Zero)  enableDBePWMxA=on  enableDBePWMxB=on  enhalfcycle=off  DBpolarity=Active high complementary (AHC)  DBedgeDelay=Positive  DBSource_ePWMxA=ePWMxA  DBSource_ePWMxB=ePWMxA  DBPeriodUnits=Clock cycles  DBperiodSource=Specify via dialog  REDperiod=5  FEDperiod=5  REDperiod_sec=0  FEDperiod_sec=0  LoadModeDBRED=Immediate without using shadow  LoadModeDBFED=Immediate without using shadow  adcstartModuleA=off  adcrequestEventA=First event  adcstartEventA=Digital Compare Module A Event 1 start of conversion (DCAEVT1.soc)  adcstartEventA_type2=Digital Compare Module A Event 1 start of conversion (DCAEVT1.soc)  adcstartModuleB=off  adcrequestEventB=First event  adcstartEventB=Counter equals to zero (CTR=Zero)  adcstartEventB_type2=Counter equals to zero (CTR=Zero)  intEn=off  intPrd=First event  intSel=Counter equals to zero (CTR=Zero)  intSel_type2=Counter equals to zero (CTR=Zero)  hrpe=off  enHRPWM=off  HRPWM_LoadMode=Counter equals to period (CTR=PRD)  HRPWM_CTLMode=Duty or Period control mode  HRPWM_EDGMode=Both edge  hrpeb=off  enHRPWMB=off  HRPWM_LoadModeB=Counter equals to zero (CTR=ZERO)  HRPWM_CTLModeB=Duty or Period control mode  HRPWM_EDGModeB=Both edge  enHRDBRED=off  enHRDBFED=off  enSFO=on  enautoconv=on  chopperEnable=off  chopperFrequency=1  chopperFirstwidth=1  chopperDuty=12.5%  tripZonesource=Specify via dialog  tzselOSHT1=off  tzselOSHT2=off  tzselOSHT3=off  tzselOSHT4=off  tzselOSHT5=off  tzselOSHT6=off  tzselOSHDCAEV1=off  tzselOSHDCBEV1=off  tzselCBC1=off  tzselCBC2=off  tzselCBC3=off  tzselCBC4=off  tzselCBC5=off  tzselCBC6=off  tzselCBCDCAEV2=off  tzselCBCDCBEV2=off  enTzOstIntr=off  enTzCbcIntr=off  enTzDCAEVT1Intr=off  enTzDCAEVT2Intr=off  enTzDCBEVT1Intr=off  enTzDCBEVT2Intr=off  tzclrCBCLatch=Counter equals to zero (CTR=Zero)  ePWMxAforced=No action  ePWMxBforced=No action  DCAEVT1forced=No action  DCBEVT1forced=No action  DCAEVT2forced=No action  DCBEVT2forced=No action  dcah=Trip Zone 1 input (TZ1)  dcal=Trip Zone 2 input (TZ2)  dcbh=Trip Zone 1 input (TZ1)  dcbl=Trip Zone 2 input (TZ2)  dcah_type2=GPTRIP1SEL/(TZ1)  dcal_type2=GPTRIP2SEL/(TZ2)  dcbh_type2=GPTRIP1SEL/(TZ1)  dcbl_type2=GPTRIP2SEL/(TZ2)  gendcaevt1=Event disabled  gendcaevt2=Event disabled  gendcbevt1=Event disabled  gendcbevt2=Event disabled  dcaevt1src=DCAEVT1 with sync  dcaevt2src=DCAEVT2 with sync  dcbevt1src=DCBEVT1 with sync  dcbevt2src=DCBEVT2 with sync  pulsesel=Counter equals to zero (CTR=Zero)  blankinv=off  blankoffset=0  blankwidth=0  evsrcsel=Filtered version of DCAEVT1 (DCAEVT1FILT)  encape=off
  ePWM6 : c2802xlib/ePWM  PwmType=C2000  useModule=ePWM6  ePWMxLINKTBPRD=Not Linked  periodUnits=Clock cycles  timerSource=Specify via dialog  timerPeriod_clk=2250  timerPeriod_sec=64000  tbshadow=Counter equals to zero  countingMode=Up-Down  phaseActiveEnable=Set counter to phase value specified via dialog  phaseDirection=Count up after sync  phaseActive=0  synchronizationEnable=off  dcaevt1Sync=off  dcbevt1Sync=off  synchronizationOption=Disable  dcbevt1SyncOut=off  dcaevt1SyncOut=off  cmpdSyncOut=off  cmpcSyncOut=off  cmpbSyncOut=off  zeroSyncOut=off  swfSyncOut=off  perSynchronizationOption=Counter equals to period (CTR=PRD)  clockPrescale=1  HSclockPrescale=1  enswap=off  ePWMxAStatus=on  ePWMxAactionLogic1=Do nothing  ePWMxAactionLogic2=Do nothing  ePWMxAactionLogic3=Clear  ePWMxAactionLogic4=Set  ePWMxAactionLogic5=Do nothing  ePWMxAactionLogic6=Do nothing  ePWMxACSFenable=off  ePWMxACSFvalue=Forcing disable  ePWMxASFreload=Zero  ePWMxBStatus=off  ePWMxBactionLogic1=Do nothing  ePWMxBactionLogic2=Set  ePWMxBactionLogic3=Do nothing  ePWMxBactionLogic4=Do nothing  ePWMxBactionLogic5=Clear  ePWMxBactionLogic6=Do nothing  ePWMxBCSFenable=off  ePWMxBCSFvalue=Forcing disable  ePWMxBSFreload=Zero  ePWNxBOutWay=off  ePWMxLINKCMPA=Not Linked  CMPAUnits=Clock cycles  CMPASource=Input port  CMPAValue_per=32000  CMPAValue_clk=floor(target.PWM_Counter_Period/2+1)  enCMPAshadow=Counter equals to zero (CTR=Zero)  ePWMxLINKCMPB=Not Linked  CMPBUnits=Clock cycles  CMPBSource=Specify via dialog  CMPBValue_per=50  CMPBValue_clk=floor(target.PWM_Counter_Period/2+1)  enCMPBshadow=Counter equals to zero (CTR=Zero)  ePWMxLINKCMPC=Not Linked  CMPCUnits=Clock cycles  CMPCSource=Specify via dialog  CMPCValue_per=50  CMPCValue_clk=32000  enCMPCshadow=Counter equals to zero (CTR=Zero)  ePWMxLINKCMPD=Not Linked  CMPDUnits=Clock cycles  CMPDSource=Specify via dialog  CMPDValue_per=50  CMPDValue_clk=32000  enCMPDshadow=Counter equals to zero (CTR=Zero)  enableDBePWMxA=on  enableDBePWMxB=on  enhalfcycle=off  DBpolarity=Active high complementary (AHC)  DBedgeDelay=Positive  DBSource_ePWMxA=ePWMxA  DBSource_ePWMxB=ePWMxA  DBPeriodUnits=Clock cycles  DBperiodSource=Specify via dialog  REDperiod=5  FEDperiod=5  REDperiod_sec=0  FEDperiod_sec=0  LoadModeDBRED=Immediate without using shadow  LoadModeDBFED=Immediate without using shadow  adcstartModuleA=off  adcrequestEventA=First event  adcstartEventA=Digital Compare Module A Event 1 start of conversion (DCAEVT1.soc)  adcstartEventA_type2=Digital Compare Module A Event 1 start of conversion (DCAEVT1.soc)  adcstartModuleB=off  adcrequestEventB=First event  adcstartEventB=Counter equals to zero (CTR=Zero)  adcstartEventB_type2=Counter equals to zero (CTR=Zero)  intEn=off  intPrd=First event  intSel=Counter equals to zero (CTR=Zero)  intSel_type2=Counter equals to zero (CTR=Zero)  hrpe=off  enHRPWM=off  HRPWM_LoadMode=Counter equals to period (CTR=PRD)  HRPWM_CTLMode=Duty or Period control mode  HRPWM_EDGMode=Both edge  hrpeb=off  enHRPWMB=off  HRPWM_LoadModeB=Counter equals to zero (CTR=ZERO)  HRPWM_CTLModeB=Duty or Period control mode  HRPWM_EDGModeB=Both edge  enHRDBRED=off  enHRDBFED=off  enSFO=on  enautoconv=on  chopperEnable=off  chopperFrequency=1  chopperFirstwidth=1  chopperDuty=12.5%  tripZonesource=Specify via dialog  tzselOSHT1=off  tzselOSHT2=off  tzselOSHT3=off  tzselOSHT4=off  tzselOSHT5=off  tzselOSHT6=off  tzselOSHDCAEV1=off  tzselOSHDCBEV1=off  tzselCBC1=off  tzselCBC2=off  tzselCBC3=off  tzselCBC4=off  tzselCBC5=off  tzselCBC6=off  tzselCBCDCAEV2=off  tzselCBCDCBEV2=off  enTzOstIntr=off  enTzCbcIntr=off  enTzDCAEVT1Intr=off  enTzDCAEVT2Intr=off  enTzDCBEVT1Intr=off  enTzDCBEVT2Intr=off  tzclrCBCLatch=Counter equals to zero (CTR=Zero)  ePWMxAforced=No action  ePWMxBforced=No action  DCAEVT1forced=No action  DCBEVT1forced=No action  DCAEVT2forced=No action  DCBEVT2forced=No action  dcah=Trip Zone 1 input (TZ1)  dcal=Trip Zone 2 input (TZ2)  dcbh=Trip Zone 1 input (TZ1)  dcbl=Trip Zone 2 input (TZ2)  dcah_type2=GPTRIP1SEL/(TZ1)  dcal_type2=GPTRIP2SEL/(TZ2)  dcbh_type2=GPTRIP1SEL/(TZ1)  dcbl_type2=GPTRIP2SEL/(TZ2)  gendcaevt1=Event disabled  gendcaevt2=Event disabled  gendcbevt1=Event disabled  gendcbevt2=Event disabled  dcaevt1src=DCAEVT1 with sync  dcaevt2src=DCAEVT2 with sync  dcbevt1src=DCBEVT1 with sync  dcbevt2src=DCBEVT2 with sync  pulsesel=Counter equals to zero (CTR=Zero)  blankinv=off  blankoffset=0  blankwidth=0  evsrcsel=Filtered version of DCAEVT1 (DCAEVT1FILT)  encape=off
  wires:
  EnPWM/1 -> Digital Output1/1
  Demux/3 -> ePWM6/1
  PWM Duty Cycle/1 -> Demux/1
  Demux/2 -> ePWM5/1
  Demux/1 -> ePWM4/1

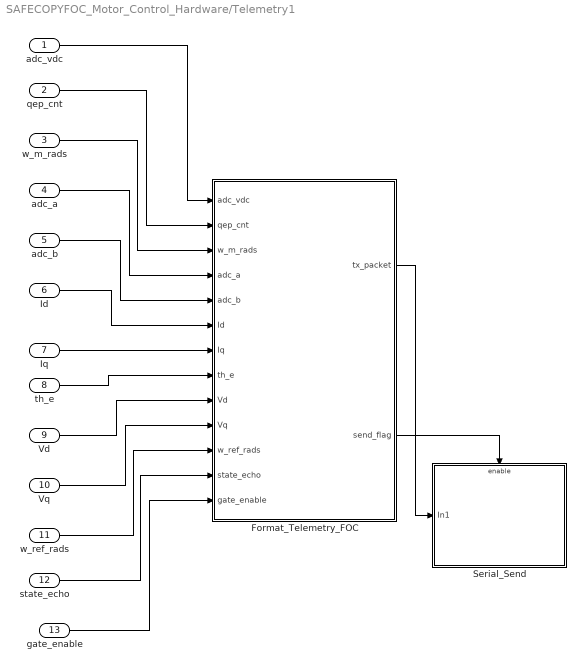
== system SAFECOPYFOC_Motor_Control_Hardware/Telemetry1 ==
  adc_vdc : Inport
  qep_cnt : Inport  Port=2
  w_m_rads : Inport  Port=3
  adc_a : Inport  Port=4
  adc_b : Inport  Port=5
  Id : Inport  Port=6
  Iq : Inport  Port=7
  th_e : Inport  Port=8
  Vd : Inport  Port=9
  Vq : Inport  Port=10
  w_ref_rads : Inport  Port=11
  state_echo : Inport  Port=12
  gate_enable : Inport  Port=13
  Format_Telemetry_FOC : MATLAB Function  TreatAsAtomicUnit=on
  Serial_Send : Subsystem  TreatAsAtomicUnit=on
  wires:
  adc_a/1 -> Format_Telemetry_FOC/4(adc_a)
  Format_Telemetry_FOC/1(tx_packet) -> Serial_Send/1(In1)
  Id/1 -> Format_Telemetry_FOC/6(Id)
  Iq/1 -> Format_Telemetry_FOC/7(Iq)
  Vd/1 -> Format_Telemetry_FOC/9(Vd)
  th_e/1 -> Format_Telemetry_FOC/8(th_e)
  w_ref_rads/1 -> Format_Telemetry_FOC/11(w_ref_rads)
  Format_Telemetry_FOC/2(send_flag) -> Serial_Send/Enable
  qep_cnt/1 -> Format_Telemetry_FOC/2(qep_cnt)
  adc_b/1 -> Format_Telemetry_FOC/5(adc_b)
  w_m_rads/1 -> Format_Telemetry_FOC/3(w_m_rads)
  Vq/1 -> Format_Telemetry_FOC/10(Vq)
  state_echo/1 -> Format_Telemetry_FOC/12(state_echo)
  gate_enable/1 -> Format_Telemetry_FOC/13(gate_enable)
  adc_vdc/1 -> Format_Telemetry_FOC/1(adc_vdc)

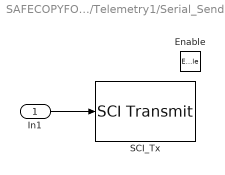
== system SAFECOPYFOC_Motor_Control_Hardware/Telemetry1/Serial_Send ==
  In1 : Inport
  Enable : EnablePort
  SCI_Tx : c280xlib/SCI Transmit  sciModule=A  dataHead=''  dataTail=''  frameSize=32  blockingMode=on  outputStatus=off
  wires:
  In1/1 -> SCI_Tx/1

== matlab function SAFECOPYFOC_Motor_Control_Hardware/Command/Decode_Command ==
function [w_ref, run_cmd, state_echo] = Decode_Command(rx_byte, calib_done)
%#codegen
persistent run_state target_w cur_state
if isempty(run_state)
    run_state = single(0);
    target_w  = single(0);
    cur_state = single(0);
end
byte = uint8(rx_byte);
if byte == uint8(49) || byte == uint8(1)      % '1' -> 100 RPM
    run_state = single(1);
    target_w  = single(10.4719755); % 100 * 2*pi/60 [rad/s]
    cur_state = single(5);         % State 5: CL FOC 100 RPM
elseif byte == uint8(50) || byte == uint8(2)  % '2' -> 200 RPM
    run_state = single(1);
    target_w  = single(20.943951);  % 200 * 2*pi/60 [rad/s]
    cur_state = single(6);         % State 6: CL FOC 200 RPM
elseif byte == uint8(48) || byte == uint8(0)  % '0' -> STOP
    run_state = single(0);
    target_w  = single(0);
    cur_state = single(0);         % State 0: STOPPED
end
if calib_done < single(0.5)
    run_cmd = single(0);
    w_ref   = single(0);
    state_echo = single(51);       % State 51: STARTUP / CALIBRATION
else
    run_cmd = run_state;
    w_ref   = target_w;
    state_echo = cur_state;
end

== matlab function SAFECOPYFOC_Motor_Control_Hardware/Feedback/Feedback_Processing ==
function [i_abc, th_e, w_m, calib_done] = Feedback_Processing(u_meas_raw, v_meas_raw, raw_qep)
%#codegen
i_abc = zeros(3, 1, 'single');
th_e = single(0);
w_m = single(0);
calib_done = single(0);
persistent offset_u offset_v calib_count cal_complete prev_th_m w_m_flt
if isempty(calib_count)
    offset_u = single(2048.0);
    offset_v = single(2048.0);
    calib_count = single(0);
    cal_complete = false;
    prev_th_m = single(0);
    w_m_flt = single(0);
end
N_CALIB = single(10000);
u_meas = single(u_meas_raw);
v_meas = single(v_meas_raw);
if ~cal_complete
    if calib_count < N_CALIB
        calib_count = calib_count + single(1.0);
        offset_u = offset_u + (u_meas - offset_u) / calib_count;
        offset_v = offset_v + (v_meas - offset_v) / calib_count;
    else
        cal_complete = true;
    end
end
K_I = single(3.3 / (4095.0 * 0.012));
i_a = (u_meas - offset_u) * K_I;
i_b = (v_meas - offset_v) * K_I;
i_c = -(i_a + i_b);
i_abc(1) = i_a;
i_abc(2) = i_b;
i_abc(3) = i_c;
TWO_PI = single(6.283185307179586);
th_m = (single(raw_qep) / single(4096.0)) * TWO_PI;
TH_OFFSET = single(1.790708);
th_e_unmod = single(21.0) * th_m + TH_OFFSET;
th_e = mod(th_e_unmod, TWO_PI);
if th_e < single(0)
    th_e = th_e + TWO_PI;
end
d_th = th_m - prev_th_m;
if d_th > single(3.14159265)
    d_th = d_th - TWO_PI;
elseif d_th < single(-3.14159265)
    d_th = d_th + TWO_PI;
end
prev_th_m = th_m;
w_m_raw = d_th * single(20000.0);
ALPHA = single(0.03);
w_m_flt = w_m_flt + ALPHA * (w_m_raw - w_m_flt);
w_m = w_m_flt;
if cal_complete
    calib_done = single(1.0);
else
    calib_done = single(0.0);
end

== matlab function SAFECOPYFOC_Motor_Control_Hardware/Telemetry1/Format_Telemetry_FOC ==
function [tx_packet, send_flag] = Format_Telemetry_FOC(adc_vdc, qep_cnt, w_m_rads, adc_a, adc_b, Id, Iq, th_e, Vd, Vq, w_ref_rads, state_echo, gate_enable)
%#codegen
persistent dec_counter
if isempty(dec_counter)
    dec_counter = single(0);
end
dec_counter = dec_counter + single(1.0);
% Decimate by 200: 20 kHz / 200 = 100 Hz serial rate
if dec_counter >= single(200.0)
    dec_counter = single(0);
    send_flag = true;
else
    send_flag = false;
end
qep_u16 = uint16(qep_cnt);
% Speed unit alignment: convert rad/s -> RPM for dashboard
spd_rpm = w_m_rads * single(9.54929658551372);
spd_i16 = typecast(int16(round(spd_rpm)), 'uint16');
adc_a_u16 = uint16(adc_a);
adc_b_u16 = uint16(adc_b);
adc_c_u16 = uint16(4096.0 - (adc_a + adc_b));
adc_vdc_u16 = uint16(adc_vdc(1));
spi_u16 = qep_u16;
Id_i16 = typecast(int16(round(max(min(Id, single(10.0)), single(-10.0)) * single(3276.7))), 'uint16');
Iq_i16 = typecast(int16(round(max(min(Iq, single(10.0)), single(-10.0)) * single(3276.7))), 'uint16');
TWO_PI = single(6.283185307179586);
theta_u16 = uint16(mod(th_e, TWO_PI) / TWO_PI * single(65535.0));
spd_cmd_rpm = w_ref_rads * single(9.54929658551372);
spd_cmd_i16 = typecast(int16(round(spd_cmd_rpm)), 'uint16');
Vd_i16 = typecast(int16(round(max(min(Vd, single(100.0)), single(-100.0)) * single(327.67))), 'uint16');
Vq_i16 = typecast(int16(round(max(min(Vq, single(100.0)), single(-100.0)) * single(327.67))), 'uint16');
tx_packet = zeros(32, 1, 'uint8');
tx_packet(1) = uint8(170);
tx_packet(2) = uint8(85);
tx_packet(3) = uint8(170);
tx_packet(4) = uint8(bitshift(qep_u16, -8));
tx_packet(5) = uint8(bitand(qep_u16, 255));
tx_packet(6) = uint8(bitshift(spd_i16, -8));
tx_packet(7) = uint8(bitand(spd_i16, 255));
tx_packet(8) = uint8(bitshift(adc_a_u16, -8));
tx_packet(9) = uint8(bitand(adc_a_u16, 255));
tx_packet(10) = uint8(bitshift(adc_b_u16, -8));
tx_packet(11) = uint8(bitand(adc_b_u16, 255));
tx_packet(12) = uint8(bitshift(adc_c_u16, -8));
tx_packet(13) = uint8(bitand(adc_c_u16, 255));
tx_packet(14) = uint8(bitshift(adc_vdc_u16, -8));
tx_packet(15) = uint8(bitand(adc_vdc_u16, 255));
tx_packet(16) = uint8(bitshift(spi_u16, -8));
tx_packet(17) = uint8(bitand(spi_u16, 255));
tx_packet(18) = uint8(bitshift(Id_i16, -8));
tx_packet(19) = uint8(bitand(Id_i16, 255));
tx_packet(20) = uint8(bitshift(Iq_i16, -8));
tx_packet(21) = uint8(bitand(Iq_i16, 255));
tx_packet(22) = uint8(bitshift(theta_u16, -8));
tx_packet(23) = uint8(bitand(theta_u16, 255));
tx_packet(24) = uint8(bitshift(spd_cmd_i16, -8));
tx_packet(25) = uint8(bitand(spd_cmd_i16, 255));
tx_packet(26) = uint8(bitshift(Vd_i16, -8));
tx_packet(27) = uint8(bitand(Vd_i16, 255));
tx_packet(28) = uint8(bitshift(Vq_i16, -8));
tx_packet(29) = uint8(bitand(Vq_i16, 255));
tx_packet(30) = uint8(state_echo);
tx_packet(31) = uint8(gate_enable);
tx_packet(32) = uint8(69);
